simulink model "modelo_FunctionalArchitecture"  (R2021b)
settings: Solver=VariableStepAuto  StartTime=0.0  StopTime=10.0  RelTol=1e-3
settings Model: Creator=The MathWorks, Inc.  LastModifiedBy=David
settings SolverCC: AlgebraicLoopSolver=TrustRegion
settings DebuggingCC: SFMachineParentedDataDiag=warning

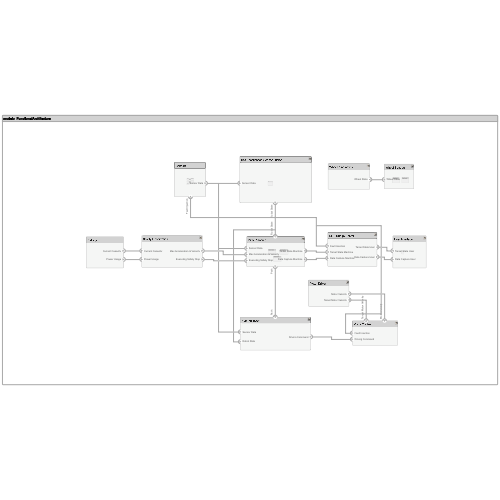
[thumbnail: Simulink's stored preview of the top-level diagram]
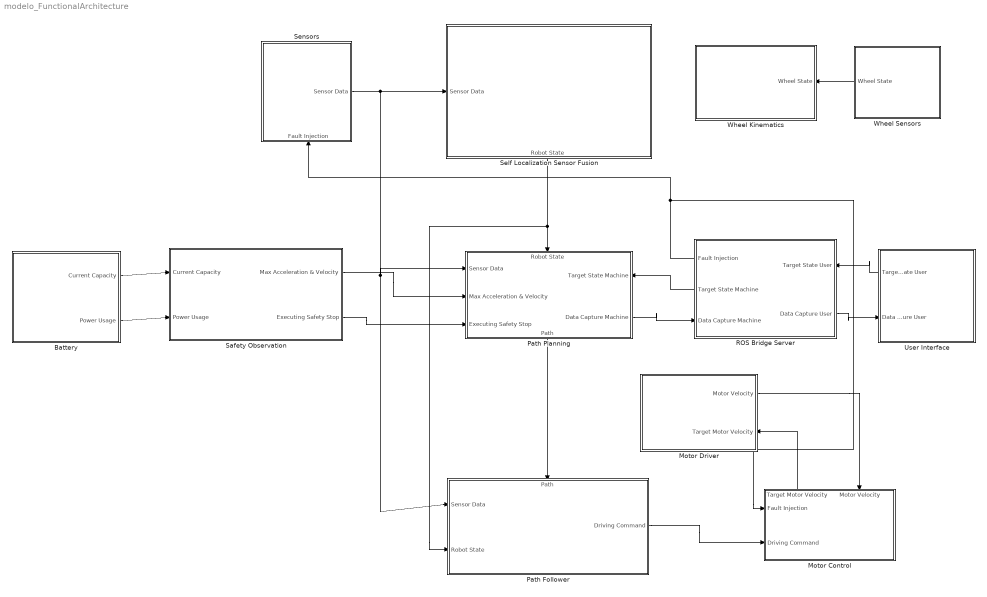
== system modelo_FunctionalArchitecture ==
  Battery : Subsystem
      settings: PortSchema="{\"entries\":[{\"content\":{\"headerSize\":26,\"margin\":15,\"minimumSpacing\":25,\"sides\":[{\"content\":{\"connectorIds\":[]},\"type\":\"ConnectorPlacement.EquallySpacedRectSide\",\"uuid\":\"59d5bf69-6351-4871-b6d0-e1e3e13a253a\"},{\"content\":{\"connectorIds\":[\"Out2\",\"Out1\"],\"side\":\"RIGHT\"},\"type\":\"ConnectorPlacement.EquallySpacedRectSide\",\"uuid\":\"4e75575f-31e6-4ae3-8223-3162d8144360\"},{\"content\":{\"connectorIds\":[],\"side\":\"TOP\"},\"type\":\"ConnectorPlacement.EquallySpacedRectSide\",\"uuid\":\"b9fd9e46-44c6-49b0-a9fa-d32b2dd616b0\"},{\"content\":{\"connectorIds\":[],\"side\":\"BOTTOM\"},\"type\":\"ConnectorPlacement.EquallySpacedRectSide\",\"uuid\":\"66421574-ce9c-483e-84db-c4bfc446eec2\"}]},\"type\":\"ConnectorPlacement.EquallySpacedConnector\",\"uuid\":\"4867c3fc-b41a-4efb-bf90-af290271d3df\"}],\"packageUris\":[\"http://schema.mathworks.com/mf0/Connector/R2020b\"],\"version\":\"1.0\"}"
  Motor Control : Subsystem
      settings: PortSchema="{\"entries\":[{\"content\":{\"headerSize\":26,\"margin\":15,\"minimumSpacing\":25,\"sides\":[{\"content\":{\"connectorIds\":[\"In1\",\"In3\"]},\"type\":\"ConnectorPlacement.EquallySpacedRectSide\",\"uuid\":\"59d5bf69-6351-4871-b6d0-e1e3e13a253a\"},{\"content\":{\"connectorIds\":[],\"side\":\"RIGHT\"},\"type\":\"ConnectorPlacement.EquallySpacedRectSide\",\"uuid\":\"4e75575f-31e6-4ae3-8223-3162d8144360\"},{\"content\":{\"connectorIds\":[\"Out1\",\"In2\"],\"side\":\"TOP\"},\"type\":\"ConnectorPlacement.EquallySpacedRectSide\",\"uuid\":\"b9fd9e46-44c6-49b0-a9fa-d32b2dd616b0\"}]},\"type\":\"ConnectorPlacement.EquallySpacedConnector\",\"uuid\":\"4867c3fc-b41a-4efb-bf90-af290271d3df\"}],\"packageUris\":[\"http://schema.mathworks.com/mf0/Connector/R2020b\"],\"version\":\"1.0\"}"
  Motor Driver : Subsystem
      settings: PortSchema="{\"entries\":[{\"content\":{\"headerSize\":26,\"margin\":15,\"minimumSpacing\":25,\"sides\":[{\"content\":{\"connectorIds\":[]},\"type\":\"ConnectorPlacement.EquallySpacedRectSide\",\"uuid\":\"59d5bf69-6351-4871-b6d0-e1e3e13a253a\"},{\"content\":{\"connectorIds\":[\"Out1\",\"In1\"],\"side\":\"RIGHT\"},\"type\":\"ConnectorPlacement.EquallySpacedRectSide\",\"uuid\":\"4e75575f-31e6-4ae3-8223-3162d8144360\"},{\"content\":{\"connectorIds\":[],\"side\":\"TOP\"},\"type\":\"ConnectorPlacement.EquallySpacedRectSide\",\"uuid\":\"b9fd9e46-44c6-49b0-a9fa-d32b2dd616b0\"},{\"content\":{\"connectorIds\":[],\"side\":\"BOTTOM\"},\"type\":\"ConnectorPlacement.EquallySpacedRectSide\",\"uuid\":\"67d81e08-878d-4ffc-8e69-7bb62ac9563c\"}]},\"type\":\"ConnectorPlacement.EquallySpacedConnector\",\"uuid\":\"4867c3fc-b41a-4efb-bf90-af290271d3df\"}],\"packageUris\":[\"http://schema.mathworks.com/mf0/Connector/R2020b\"],\"version\":\"1.0\"}"
  Path Follower : Subsystem
      settings: PortSchema="{\"entries\":[{\"content\":{\"headerSize\":26,\"margin\":15,\"minimumSpacing\":25,\"sides\":[{\"content\":{\"connectorIds\":[\"In1\",\"In3\"]},\"type\":\"ConnectorPlacement.EquallySpacedRectSide\",\"uuid\":\"59d5bf69-6351-4871-b6d0-e1e3e13a253a\"},{\"content\":{\"connectorIds\":[\"Out1\"],\"side\":\"RIGHT\"},\"type\":\"ConnectorPlacement.EquallySpacedRectSide\",\"uuid\":\"4e75575f-31e6-4ae3-8223-3162d8144360\"},{\"content\":{\"connectorIds\":[\"In2\"],\"side\":\"TOP\"},\"type\":\"ConnectorPlacement.EquallySpacedRectSide\",\"uuid\":\"b9fd9e46-44c6-49b0-a9fa-d32b2dd616b0\"}]},\"type\":\"ConnectorPlacement.EquallySpacedConnector\",\"uuid\":\"4867c3fc-b41a-4efb-bf90-af290271d3df\"}],\"packageUris\":[\"http://schema.mathworks.com/mf0/Connector/R2020b\"],\"version\":\"1.0\"}"
  Path Planning : Subsystem
      settings: PortSchema="{\"entries\":[{\"content\":{\"headerSize\":26,\"margin\":15,\"minimumSpacing\":25,\"sides\":[{\"content\":{\"connectorIds\":[\"In1\",\"In2\",\"In3\"]},\"type\":\"ConnectorPlacement.EquallySpacedRectSide\",\"uuid\":\"59d5bf69-6351-4871-b6d0-e1e3e13a253a\"},{\"content\":{\"connectorIds\":[\"In4\",\"Out1\"],\"side\":\"RIGHT\"},\"type\":\"ConnectorPlacement.EquallySpacedRectSide\",\"uuid\":\"4e75575f-31e6-4ae3-8223-3162d8144360\"},{\"content\":{\"connectorIds\":[\"In5\"],\"side\":\"TOP\"},\"type\":\"ConnectorPlacement.EquallySpacedRectSide\",\"uuid\":\"b9fd9e46-44c6-49b0-a9fa-d32b2dd616b0\"},{\"content\":{\"connectorIds\":[\"Out2\"],\"side\":\"BOTTOM\"},\"type\":\"ConnectorPlacement.EquallySpacedRectSide\",\"uuid\":\"b63bab7c-787a-46d6-b750-862a2a39c4b0\"}]},\"type\":\"ConnectorPlacement.EquallySpacedConnector\",\"uuid\":\"4867c3fc-b41a-4efb-bf90-af290271d3df\"}],\"packageUris\":[\"http://schema.mathworks.com/mf0/Connector/R2020b\"],\"version\":\"1.0\"}"
  ROS Bridge Server : Subsystem
      settings: PortSchema="{\"entries\":[{\"content\":{\"headerSize\":26,\"margin\":15,\"minimumSpacing\":25,\"sides\":[{\"content\":{\"connectorIds\":[\"Out1\",\"Out3\",\"In1\"]},\"type\":\"ConnectorPlacement.EquallySpacedRectSide\",\"uuid\":\"78ec9596-c19b-4a19-90cc-d79d904dcecb\"},{\"content\":{\"connectorIds\":[\"In2\",\"Out2\"],\"side\":\"RIGHT\"},\"type\":\"ConnectorPlacement.EquallySpacedRectSide\",\"uuid\":\"e50c32f8-61a1-4c3e-810e-7c092ec61b9d\"},{\"content\":{\"connectorIds\":[],\"side\":\"TOP\"},\"type\":\"ConnectorPlacement.EquallySpacedRectSide\",\"uuid\":\"dd5589de-c446-44bc-b6c3-43d178c94f81\"}]},\"type\":\"ConnectorPlacement.EquallySpacedConnector\",\"uuid\":\"1e9f716a-1f22-4423-b94e-8264810d47f5\"}],\"packageUris\":[\"http://schema.mathworks.com/mf0/Connector/R2020b\"],\"version\":\"1.0\"}"
  Safety Observation : Subsystem
      settings: PortSchema="{\"entries\":[{\"content\":{\"headerSize\":26,\"margin\":15,\"minimumSpacing\":25,\"sides\":[{\"content\":{\"connectorIds\":[\"In2\",\"In1\"]},\"type\":\"ConnectorPlacement.EquallySpacedRectSide\",\"uuid\":\"59d5bf69-6351-4871-b6d0-e1e3e13a253a\"},{\"content\":{\"connectorIds\":[\"Out2\",\"Out1\"],\"side\":\"RIGHT\"},\"type\":\"ConnectorPlacement.EquallySpacedRectSide\",\"uuid\":\"4e75575f-31e6-4ae3-8223-3162d8144360\"},{\"content\":{\"connectorIds\":[],\"side\":\"TOP\"},\"type\":\"ConnectorPlacement.EquallySpacedRectSide\",\"uuid\":\"b9fd9e46-44c6-49b0-a9fa-d32b2dd616b0\"},{\"content\":{\"connectorIds\":[],\"side\":\"BOTTOM\"},\"type\":\"ConnectorPlacement.EquallySpacedRectSide\",\"uuid\":\"4263e838-8ece-4353-a266-fb02fc9beff8\"}]},\"type\":\"ConnectorPlacement.EquallySpacedConnector\",\"uuid\":\"4867c3fc-b41a-4efb-bf90-af290271d3df\"}],\"packageUris\":[\"http://schema.mathworks.com/mf0/Connector/R2020b\"],\"version\":\"1.0\"}"
  Self Localization Sensor Fusion : Subsystem
      settings: PortSchema="{\"entries\":[{\"content\":{\"headerSize\":26,\"margin\":15,\"minimumSpacing\":25,\"sides\":[{\"content\":{\"connectorIds\":[\"In1\"]},\"type\":\"ConnectorPlacement.EquallySpacedRectSide\",\"uuid\":\"59d5bf69-6351-4871-b6d0-e1e3e13a253a\"},{\"content\":{\"connectorIds\":[],\"side\":\"RIGHT\"},\"type\":\"ConnectorPlacement.EquallySpacedRectSide\",\"uuid\":\"4e75575f-31e6-4ae3-8223-3162d8144360\"},{\"content\":{\"connectorIds\":[],\"side\":\"TOP\"},\"type\":\"ConnectorPlacement.EquallySpacedRectSide\",\"uuid\":\"b9fd9e46-44c6-49b0-a9fa-d32b2dd616b0\"},{\"content\":{\"connectorIds\":[\"Out1\"],\"side\":\"BOTTOM\"},\"type\":\"ConnectorPlacement.EquallySpacedRectSide\",\"uuid\":\"114bac9a-6c92-45bb-ae46-c4bda2c799d1\"}]},\"type\":\"ConnectorPlacement.EquallySpacedConnector\",\"uuid\":\"4867c3fc-b41a-4efb-bf90-af290271d3df\"}],\"packageUris\":[\"http://schema.mathworks.com/mf0/Connector/R2020b\"],\"version\":\"1.0\"}"
  Sensors : Subsystem
      settings: PortSchema="{\"entries\":[{\"content\":{\"headerSize\":26,\"margin\":15,\"minimumSpacing\":25,\"sides\":[{\"content\":{\"connectorIds\":[]},\"type\":\"ConnectorPlacement.EquallySpacedRectSide\",\"uuid\":\"78ec9596-c19b-4a19-90cc-d79d904dcecb\"},{\"content\":{\"connectorIds\":[\"Out1\"],\"side\":\"RIGHT\"},\"type\":\"ConnectorPlacement.EquallySpacedRectSide\",\"uuid\":\"e50c32f8-61a1-4c3e-810e-7c092ec61b9d\"},{\"content\":{\"connectorIds\":[],\"side\":\"TOP\"},\"type\":\"ConnectorPlacement.EquallySpacedRectSide\",\"uuid\":\"dd5589de-c446-44bc-b6c3-43d178c94f81\"},{\"content\":{\"connectorIds\":[\"In1\"],\"side\":\"BOTTOM\"},\"type\":\"ConnectorPlacement.EquallySpacedRectSide\",\"uuid\":\"022d1208-42d8-4ed3-aa9f-a16a2de5d603\"}]},\"type\":\"ConnectorPlacement.EquallySpacedConnector\",\"uuid\":\"1e9f716a-1f22-4423-b94e-8264810d47f5\"}],\"packageUris\":[\"http://schema.mathworks.com/mf0/Connector/R2020b\"],\"version\":\"1.0\"}"
  User Interface : Subsystem
      settings: PortSchema="{\"entries\":[{\"content\":{\"headerSize\":26,\"margin\":15,\"minimumSpacing\":25,\"sides\":[{\"content\":{\"connectorIds\":[\"Out1\",\"In1\"]},\"type\":\"ConnectorPlacement.EquallySpacedRectSide\",\"uuid\":\"59d5bf69-6351-4871-b6d0-e1e3e13a253a\"},{\"content\":{\"connectorIds\":[],\"side\":\"RIGHT\"},\"type\":\"ConnectorPlacement.EquallySpacedRectSide\",\"uuid\":\"4e75575f-31e6-4ae3-8223-3162d8144360\"},{\"content\":{\"connectorIds\":[],\"side\":\"TOP\"},\"type\":\"ConnectorPlacement.EquallySpacedRectSide\",\"uuid\":\"b9fd9e46-44c6-49b0-a9fa-d32b2dd616b0\"},{\"content\":{\"connectorIds\":[],\"side\":\"BOTTOM\"},\"type\":\"ConnectorPlacement.EquallySpacedRectSide\",\"uuid\":\"51492fe5-00fa-4995-98e1-4969e22079d3\"}]},\"type\":\"ConnectorPlacement.EquallySpacedConnector\",\"uuid\":\"4867c3fc-b41a-4efb-bf90-af290271d3df\"}],\"packageUris\":[\"http://schema.mathworks.com/mf0/Connector/R2020b\"],\"version\":\"1.0\"}"
  Wheel Kinematics : Subsystem
      settings: PortSchema="{\"entries\":[{\"content\":{\"headerSize\":26,\"margin\":15,\"minimumSpacing\":25,\"sides\":[{\"content\":{\"connectorIds\":[]},\"type\":\"ConnectorPlacement.EquallySpacedRectSide\",\"uuid\":\"8b00e6c1-78bc-425f-98b4-5345e91b6ef3\"},{\"content\":{\"connectorIds\":[\"In1\"],\"side\":\"RIGHT\"},\"type\":\"ConnectorPlacement.EquallySpacedRectSide\",\"uuid\":\"cca7f40b-c9e3-40f8-88e3-c95e453373a7\"},{\"content\":{\"connectorIds\":[],\"side\":\"TOP\"},\"type\":\"ConnectorPlacement.EquallySpacedRectSide\",\"uuid\":\"2cebc568-363b-44c7-85e9-8321d53d58f8\"}]},\"type\":\"ConnectorPlacement.EquallySpacedConnector\",\"uuid\":\"893f8d0c-b80d-487c-8abd-26601278087d\"}],\"packageUris\":[\"http://schema.mathworks.com/mf0/Connector/R2020b\"],\"version\":\"1.0\"}"
  Wheel Sensors : Subsystem
      settings: PortSchema="{\"entries\":[{\"content\":{\"headerSize\":26,\"margin\":15,\"minimumSpacing\":25,\"sides\":[{\"content\":{\"connectorIds\":[\"Out1\"]},\"type\":\"ConnectorPlacement.EquallySpacedRectSide\",\"uuid\":\"59d5bf69-6351-4871-b6d0-e1e3e13a253a\"},{\"content\":{\"connectorIds\":[],\"side\":\"RIGHT\"},\"type\":\"ConnectorPlacement.EquallySpacedRectSide\",\"uuid\":\"4e75575f-31e6-4ae3-8223-3162d8144360\"},{\"content\":{\"connectorIds\":[],\"side\":\"TOP\"},\"type\":\"ConnectorPlacement.EquallySpacedRectSide\",\"uuid\":\"b9fd9e46-44c6-49b0-a9fa-d32b2dd616b0\"}]},\"type\":\"ConnectorPlacement.EquallySpacedConnector\",\"uuid\":\"4867c3fc-b41a-4efb-bf90-af290271d3df\"}],\"packageUris\":[\"http://schema.mathworks.com/mf0/Connector/R2020b\"],\"version\":\"1.0\"}"
  wires:
  Self Localization Sensor Fusion/1(Robot State) -> Path Follower/3(Robot State), Path Planning/5(Robot State)
  Safety Observation/2(Max Acceleration & Velocity) -> Path Planning/2(Max Acceleration & Velocity)
  Path Follower/1(Driving Command) -> Motor Control/3(Driving Command)
  Battery/1(Power Usage) -> Safety Observation/1(Power Usage)
  Battery/2(Current Capacity) -> Safety Observation/2(Current Capacity)
  Motor Driver/1(Motor Velocity) -> Motor Control/2(Motor Velocity)
  Motor Control/1(Target Motor Velocity) -> Motor Driver/1(Target Motor Velocity)
  Path Planning/2(Path) -> Path Follower/2(Path)
  Safety Observation/1(Executing Safety Stop) -> Path Planning/3(Executing Safety Stop)
  Wheel Sensors/1(Wheel State) -> Wheel Kinematics/1(Wheel State)
  User Interface/1(Target State User) -> ROS Bridge Server/2(Target State User)
  ROS Bridge Server/3(Target State Machine) -> Path Planning/4(Target State Machine)
  Path Planning/1(Data Capture Machine) -> ROS Bridge Server/1(Data Capture Machine)
  ROS Bridge Server/2(Data Capture User) -> User Interface/1(Data Capture User)
  Sensors/1(Sensor Data) -> Path Follower/1(Sensor Data), Path Planning/1(Sensor Data), Self Localization Sensor Fusion/1(Sensor Data)
  ROS Bridge Server/1(Fault Injection) -> Motor Control/1(Fault Injection), Sensors/1(Fault Injection)

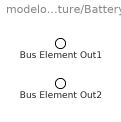
== system modelo_FunctionalArchitecture/Battery ==
  Bus Element Out1 : Outport  PortName=Power Usage
  Bus Element Out2 : Outport  Port=2  PortName=Current Capacity

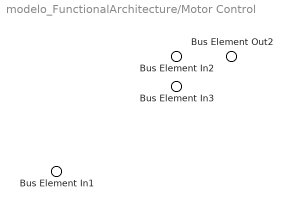
== system modelo_FunctionalArchitecture/Motor Control ==
  Bus Element In3 : Inport  PortName=Fault Injection
  Bus Element In2 : Inport  Port=2  PortName=Motor Velocity
  Bus Element In1 : Inport  Port=3  PortName=Driving Command
  Bus Element Out2 : Outport  PortName=Target Motor Velocity

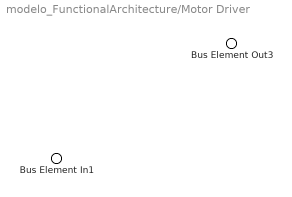
== system modelo_FunctionalArchitecture/Motor Driver ==
  Bus Element In1 : Inport  PortName=Target Motor Velocity
  Bus Element Out3 : Outport  PortName=Motor Velocity

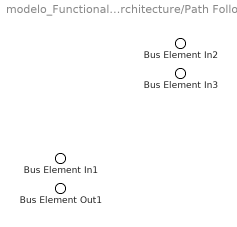
== system modelo_FunctionalArchitecture/Path Follower ==
  Bus Element In2 : Inport  PortName=Sensor Data
  Bus Element In3 : Inport  Port=2  PortName=Path
  Bus Element In1 : Inport  Port=3  PortName=Robot State
  Bus Element Out1 : Outport  PortName=Driving Command

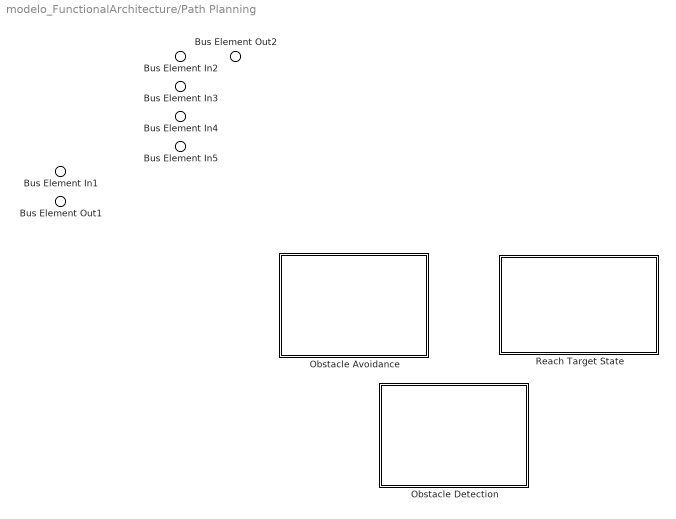
== system modelo_FunctionalArchitecture/Path Planning ==
  Bus Element In3 : Inport  PortName=Sensor Data
  Bus Element In4 : Inport  Port=2  PortName=Max Acceleration & Velocity
  Bus Element In5 : Inport  Port=3  PortName=Executing Safety Stop
  Bus Element In2 : Inport  Port=4  PortName=Target State Machine
  Bus Element In1 : Inport  Port=5  PortName=Robot State
  Obstacle Avoidance : Subsystem
      settings: PortSchema="{\"entries\":[{\"content\":{\"headerSize\":26,\"margin\":15,\"minimumSpacing\":25,\"sides\":[{\"content\":{\"connectorIds\":[]},\"type\":\"ConnectorPlacement.EquallySpacedRectSide\",\"uuid\":\"623c0a04-b13a-4ec6-8a7d-dfc6306469bc\"},{\"content\":{\"connectorIds\":[],\"side\":\"RIGHT\"},\"type\":\"ConnectorPlacement.EquallySpacedRectSide\",\"uuid\":\"78f920bb-0077-4b2a-aa3f-2f201c60998f\"},{\"content\":{\"connectorIds\":[],\"side\":\"TOP\"},\"type\":\"ConnectorPlacement.EquallySpacedRectSide\",\"uuid\":\"9b1e3f50-ee79-4c39-a86a-2d702aea3294\"},{\"content\":{\"connectorIds\":[],\"side\":\"HIDDEN\"},\"type\":\"ConnectorPlacement.EquallySpacedRectSide\",\"uuid\":\"cdf686db-25c9-46dd-b452-4d2a5526d98f\"}]},\"type\":\"ConnectorPlacement.EquallySpacedConnector\",\"uuid\":\"0b3e7296-fe8f-4ed3-b294-7805e2066d7f\"}],\"packageUris\":[\"http://schema.mathworks.com/mf0/Connector/R2020b\"],\"version\":\"1.0\"}"
  Obstacle Detection : Subsystem
      settings: PortSchema="{\"entries\":[{\"content\":{\"headerSize\":26,\"margin\":15,\"minimumSpacing\":25,\"sides\":[{\"content\":{\"connectorIds\":[]},\"type\":\"ConnectorPlacement.EquallySpacedRectSide\",\"uuid\":\"623c0a04-b13a-4ec6-8a7d-dfc6306469bc\"},{\"content\":{\"connectorIds\":[],\"side\":\"RIGHT\"},\"type\":\"ConnectorPlacement.EquallySpacedRectSide\",\"uuid\":\"78f920bb-0077-4b2a-aa3f-2f201c60998f\"},{\"content\":{\"connectorIds\":[],\"side\":\"TOP\"},\"type\":\"ConnectorPlacement.EquallySpacedRectSide\",\"uuid\":\"9b1e3f50-ee79-4c39-a86a-2d702aea3294\"},{\"content\":{\"connectorIds\":[],\"side\":\"HIDDEN\"},\"type\":\"ConnectorPlacement.EquallySpacedRectSide\",\"uuid\":\"cdf686db-25c9-46dd-b452-4d2a5526d98f\"}]},\"type\":\"ConnectorPlacement.EquallySpacedConnector\",\"uuid\":\"0b3e7296-fe8f-4ed3-b294-7805e2066d7f\"}],\"packageUris\":[\"http://schema.mathworks.com/mf0/Connector/R2020b\"],\"version\":\"1.0\"}"
  Reach Target State : Subsystem
      settings: PortSchema="{\"entries\":[{\"content\":{\"headerSize\":26,\"margin\":15,\"minimumSpacing\":25,\"sides\":[{\"content\":{\"connectorIds\":[]},\"type\":\"ConnectorPlacement.EquallySpacedRectSide\",\"uuid\":\"623c0a04-b13a-4ec6-8a7d-dfc6306469bc\"},{\"content\":{\"connectorIds\":[],\"side\":\"RIGHT\"},\"type\":\"ConnectorPlacement.EquallySpacedRectSide\",\"uuid\":\"78f920bb-0077-4b2a-aa3f-2f201c60998f\"},{\"content\":{\"connectorIds\":[],\"side\":\"TOP\"},\"type\":\"ConnectorPlacement.EquallySpacedRectSide\",\"uuid\":\"9b1e3f50-ee79-4c39-a86a-2d702aea3294\"},{\"content\":{\"connectorIds\":[],\"side\":\"HIDDEN\"},\"type\":\"ConnectorPlacement.EquallySpacedRectSide\",\"uuid\":\"cdf686db-25c9-46dd-b452-4d2a5526d98f\"}]},\"type\":\"ConnectorPlacement.EquallySpacedConnector\",\"uuid\":\"0b3e7296-fe8f-4ed3-b294-7805e2066d7f\"}],\"packageUris\":[\"http://schema.mathworks.com/mf0/Connector/R2020b\"],\"version\":\"1.0\"}"
  Bus Element Out2 : Outport  PortName=Data Capture Machine
  Bus Element Out1 : Outport  Port=2  PortName=Path

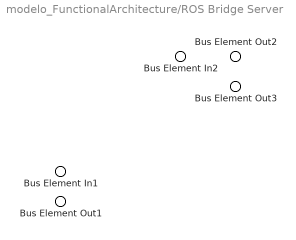
== system modelo_FunctionalArchitecture/ROS Bridge Server ==
  Bus Element In2 : Inport  PortName=Data Capture Machine
  Bus Element In1 : Inport  Port=2  PortName=Target State User
  Bus Element Out3 : Outport  PortName=Fault Injection
  Bus Element Out2 : Outport  Port=2  PortName=Data Capture User
  Bus Element Out1 : Outport  Port=3  PortName=Target State Machine

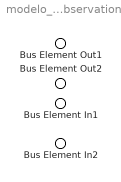
== system modelo_FunctionalArchitecture/Safety Observation ==
  Bus Element In1 : Inport  PortName=Power Usage
  Bus Element In2 : Inport  Port=2  PortName=Current Capacity
  Bus Element Out1 : Outport  PortName=Executing Safety Stop
  Bus Element Out2 : Outport  Port=2  PortName=Max Acceleration & Velocity

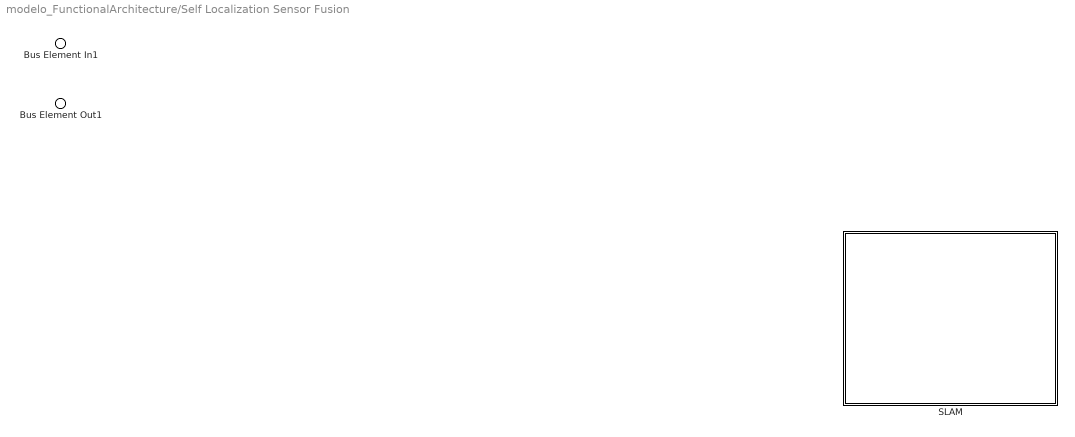
== system modelo_FunctionalArchitecture/Self Localization Sensor Fusion ==
  Bus Element In1 : Inport  PortName=Sensor Data
  SLAM : Subsystem
      settings: PortSchema="{\"entries\":[{\"content\":{\"headerSize\":26,\"margin\":15,\"minimumSpacing\":25,\"sides\":[{\"content\":{\"connectorIds\":[]},\"type\":\"ConnectorPlacement.EquallySpacedRectSide\",\"uuid\":\"78ec9596-c19b-4a19-90cc-d79d904dcecb\"},{\"content\":{\"connectorIds\":[],\"side\":\"RIGHT\"},\"type\":\"ConnectorPlacement.EquallySpacedRectSide\",\"uuid\":\"e50c32f8-61a1-4c3e-810e-7c092ec61b9d\"},{\"content\":{\"connectorIds\":[],\"side\":\"TOP\"},\"type\":\"ConnectorPlacement.EquallySpacedRectSide\",\"uuid\":\"dd5589de-c446-44bc-b6c3-43d178c94f81\"}]},\"type\":\"ConnectorPlacement.EquallySpacedConnector\",\"uuid\":\"1e9f716a-1f22-4423-b94e-8264810d47f5\"}],\"packageUris\":[\"http://schema.mathworks.com/mf0/Connector/R2020b\"],\"version\":\"1.0\"}"
  Bus Element Out1 : Outport  PortName=Robot State

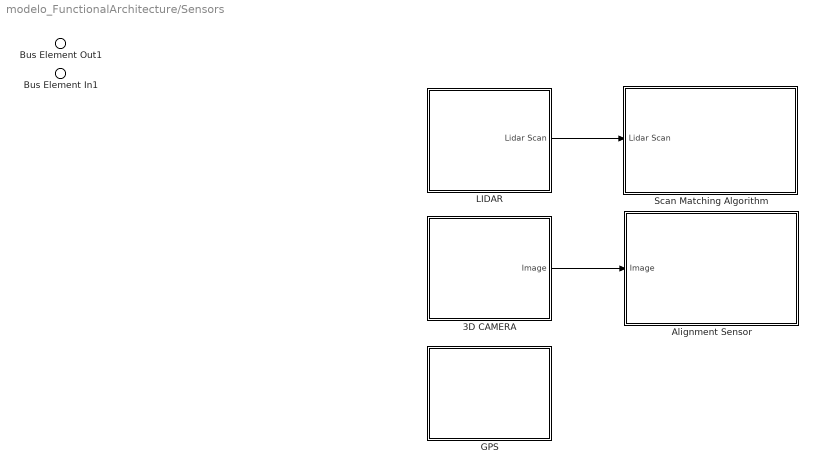
== system modelo_FunctionalArchitecture/Sensors ==
  Bus Element In1 : Inport  PortName=Fault Injection
  3D CAMERA : Subsystem
      settings: PortSchema="{\"entries\":[{\"content\":{\"headerSize\":26,\"margin\":15,\"minimumSpacing\":25,\"sides\":[{\"content\":{\"connectorIds\":[]},\"type\":\"ConnectorPlacement.EquallySpacedRectSide\",\"uuid\":\"8b00e6c1-78bc-425f-98b4-5345e91b6ef3\"},{\"content\":{\"connectorIds\":[\"Out1\"],\"side\":\"RIGHT\"},\"type\":\"ConnectorPlacement.EquallySpacedRectSide\",\"uuid\":\"cca7f40b-c9e3-40f8-88e3-c95e453373a7\"},{\"content\":{\"connectorIds\":[],\"side\":\"TOP\"},\"type\":\"ConnectorPlacement.EquallySpacedRectSide\",\"uuid\":\"2cebc568-363b-44c7-85e9-8321d53d58f8\"}]},\"type\":\"ConnectorPlacement.EquallySpacedConnector\",\"uuid\":\"893f8d0c-b80d-487c-8abd-26601278087d\"}],\"packageUris\":[\"http://schema.mathworks.com/mf0/Connector/R2020b\"],\"version\":\"1.0\"}"
  Alignment Sensor : Subsystem
      settings: PortSchema="{\"entries\":[{\"content\":{\"headerSize\":26,\"margin\":15,\"minimumSpacing\":25,\"sides\":[{\"content\":{\"connectorIds\":[\"In1\"]},\"type\":\"ConnectorPlacement.EquallySpacedRectSide\",\"uuid\":\"8b00e6c1-78bc-425f-98b4-5345e91b6ef3\"},{\"content\":{\"connectorIds\":[],\"side\":\"RIGHT\"},\"type\":\"ConnectorPlacement.EquallySpacedRectSide\",\"uuid\":\"cca7f40b-c9e3-40f8-88e3-c95e453373a7\"},{\"content\":{\"connectorIds\":[],\"side\":\"TOP\"},\"type\":\"ConnectorPlacement.EquallySpacedRectSide\",\"uuid\":\"2cebc568-363b-44c7-85e9-8321d53d58f8\"}]},\"type\":\"ConnectorPlacement.EquallySpacedConnector\",\"uuid\":\"893f8d0c-b80d-487c-8abd-26601278087d\"}],\"packageUris\":[\"http://schema.mathworks.com/mf0/Connector/R2020b\"],\"version\":\"1.0\"}"
  GPS : Subsystem
      settings: PortSchema="{\"entries\":[{\"content\":{\"headerSize\":26,\"margin\":15,\"minimumSpacing\":25,\"sides\":[{\"content\":{\"connectorIds\":[]},\"type\":\"ConnectorPlacement.EquallySpacedRectSide\",\"uuid\":\"78ec9596-c19b-4a19-90cc-d79d904dcecb\"},{\"content\":{\"connectorIds\":[],\"side\":\"RIGHT\"},\"type\":\"ConnectorPlacement.EquallySpacedRectSide\",\"uuid\":\"e50c32f8-61a1-4c3e-810e-7c092ec61b9d\"},{\"content\":{\"connectorIds\":[],\"side\":\"TOP\"},\"type\":\"ConnectorPlacement.EquallySpacedRectSide\",\"uuid\":\"dd5589de-c446-44bc-b6c3-43d178c94f81\"}]},\"type\":\"ConnectorPlacement.EquallySpacedConnector\",\"uuid\":\"1e9f716a-1f22-4423-b94e-8264810d47f5\"}],\"packageUris\":[\"http://schema.mathworks.com/mf0/Connector/R2020b\"],\"version\":\"1.0\"}"
  LIDAR : Subsystem
      settings: PortSchema="{\"entries\":[{\"content\":{\"headerSize\":26,\"margin\":15,\"minimumSpacing\":25,\"sides\":[{\"content\":{\"connectorIds\":[]},\"type\":\"ConnectorPlacement.EquallySpacedRectSide\",\"uuid\":\"59d5bf69-6351-4871-b6d0-e1e3e13a253a\"},{\"content\":{\"connectorIds\":[\"Out1\"],\"side\":\"RIGHT\"},\"type\":\"ConnectorPlacement.EquallySpacedRectSide\",\"uuid\":\"4e75575f-31e6-4ae3-8223-3162d8144360\"},{\"content\":{\"connectorIds\":[],\"side\":\"TOP\"},\"type\":\"ConnectorPlacement.EquallySpacedRectSide\",\"uuid\":\"b9fd9e46-44c6-49b0-a9fa-d32b2dd616b0\"}]},\"type\":\"ConnectorPlacement.EquallySpacedConnector\",\"uuid\":\"4867c3fc-b41a-4efb-bf90-af290271d3df\"}],\"packageUris\":[\"http://schema.mathworks.com/mf0/Connector/R2020b\"],\"version\":\"1.0\"}"
  Scan Matching Algorithm : Subsystem
      settings: PortSchema="{\"entries\":[{\"content\":{\"headerSize\":26,\"margin\":15,\"minimumSpacing\":25,\"sides\":[{\"content\":{\"connectorIds\":[\"In1\"]},\"type\":\"ConnectorPlacement.EquallySpacedRectSide\",\"uuid\":\"8b00e6c1-78bc-425f-98b4-5345e91b6ef3\"},{\"content\":{\"connectorIds\":[],\"side\":\"RIGHT\"},\"type\":\"ConnectorPlacement.EquallySpacedRectSide\",\"uuid\":\"cca7f40b-c9e3-40f8-88e3-c95e453373a7\"},{\"content\":{\"connectorIds\":[],\"side\":\"TOP\"},\"type\":\"ConnectorPlacement.EquallySpacedRectSide\",\"uuid\":\"2cebc568-363b-44c7-85e9-8321d53d58f8\"}]},\"type\":\"ConnectorPlacement.EquallySpacedConnector\",\"uuid\":\"893f8d0c-b80d-487c-8abd-26601278087d\"}],\"packageUris\":[\"http://schema.mathworks.com/mf0/Connector/R2020b\"],\"version\":\"1.0\"}"
  Bus Element Out1 : Outport  PortName=Sensor Data
  wires:
  3D CAMERA/1(Image) -> Alignment Sensor/1(Image)
  LIDAR/1(Lidar Scan) -> Scan Matching Algorithm/1(Lidar Scan)

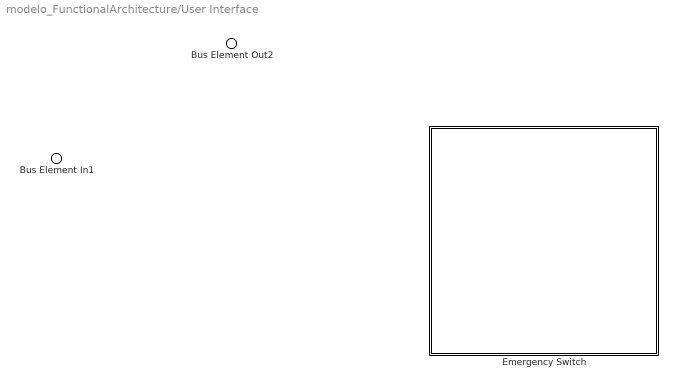
== system modelo_FunctionalArchitecture/User Interface ==
  Bus Element In1 : Inport  PortName=Data Capture User
  Emergency Switch : Subsystem
      settings: PortSchema="{\"entries\":[{\"content\":{\"headerSize\":26,\"margin\":15,\"minimumSpacing\":25,\"sides\":[{\"content\":{\"connectorIds\":[]},\"type\":\"ConnectorPlacement.EquallySpacedRectSide\",\"uuid\":\"78ec9596-c19b-4a19-90cc-d79d904dcecb\"},{\"content\":{\"connectorIds\":[],\"side\":\"RIGHT\"},\"type\":\"ConnectorPlacement.EquallySpacedRectSide\",\"uuid\":\"e50c32f8-61a1-4c3e-810e-7c092ec61b9d\"},{\"content\":{\"connectorIds\":[],\"side\":\"TOP\"},\"type\":\"ConnectorPlacement.EquallySpacedRectSide\",\"uuid\":\"dd5589de-c446-44bc-b6c3-43d178c94f81\"}]},\"type\":\"ConnectorPlacement.EquallySpacedConnector\",\"uuid\":\"1e9f716a-1f22-4423-b94e-8264810d47f5\"}],\"packageUris\":[\"http://schema.mathworks.com/mf0/Connector/R2020b\"],\"version\":\"1.0\"}"
  Bus Element Out2 : Outport  PortName=Target State User

== system modelo_FunctionalArchitecture/Wheel Kinematics ==
  Bus Element In1 : Inport  PortName=Wheel State

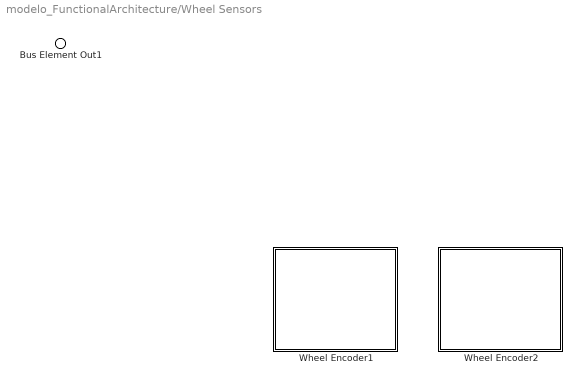
== system modelo_FunctionalArchitecture/Wheel Sensors ==
  Wheel Encoder1 : Subsystem
      settings: PortSchema="{\"entries\":[{\"content\":{\"headerSize\":26,\"margin\":15,\"minimumSpacing\":25,\"sides\":[{\"content\":{\"connectorIds\":[]},\"type\":\"ConnectorPlacement.EquallySpacedRectSide\",\"uuid\":\"6da287f1-0145-4984-81ce-516f9d473d08\"},{\"content\":{\"connectorIds\":[],\"side\":\"RIGHT\"},\"type\":\"ConnectorPlacement.EquallySpacedRectSide\",\"uuid\":\"e8258003-a16e-4667-bad1-2432c305b2b4\"},{\"content\":{\"connectorIds\":[],\"side\":\"TOP\"},\"type\":\"ConnectorPlacement.EquallySpacedRectSide\",\"uuid\":\"774c20e3-3d70-4446-b47a-ebbe701b6bb4\"}]},\"type\":\"ConnectorPlacement.EquallySpacedConnector\",\"uuid\":\"18cfb653-cd4a-4ba6-a2cf-b79d05bb2a8a\"}],\"packageUris\":[\"http://schema.mathworks.com/mf0/Connector/R2020b\"],\"version\":\"1.0\"}"
  Wheel Encoder2 : Subsystem
      settings: PortSchema="{\"entries\":[{\"content\":{\"headerSize\":26,\"margin\":15,\"minimumSpacing\":25,\"sides\":[{\"content\":{\"connectorIds\":[]},\"type\":\"ConnectorPlacement.EquallySpacedRectSide\",\"uuid\":\"6da287f1-0145-4984-81ce-516f9d473d08\"},{\"content\":{\"connectorIds\":[],\"side\":\"RIGHT\"},\"type\":\"ConnectorPlacement.EquallySpacedRectSide\",\"uuid\":\"e8258003-a16e-4667-bad1-2432c305b2b4\"},{\"content\":{\"connectorIds\":[],\"side\":\"TOP\"},\"type\":\"ConnectorPlacement.EquallySpacedRectSide\",\"uuid\":\"774c20e3-3d70-4446-b47a-ebbe701b6bb4\"}]},\"type\":\"ConnectorPlacement.EquallySpacedConnector\",\"uuid\":\"18cfb653-cd4a-4ba6-a2cf-b79d05bb2a8a\"}],\"packageUris\":[\"http://schema.mathworks.com/mf0/Connector/R2020b\"],\"version\":\"1.0\"}"
  Bus Element Out1 : Outport  PortName=Wheel State

== system modelo_FunctionalArchitecture/Path Planning/Obstacle Avoidance ==

== system modelo_FunctionalArchitecture/Path Planning/Obstacle Detection ==

== system modelo_FunctionalArchitecture/Path Planning/Reach Target State ==

== system modelo_FunctionalArchitecture/Self Localization Sensor Fusion/SLAM ==

== system modelo_FunctionalArchitecture/Sensors/3D CAMERA ==
  Bus Element Out1 : Outport  PortName=Image

== system modelo_FunctionalArchitecture/Sensors/Alignment Sensor ==
  Bus Element In1 : Inport  PortName=Image

== system modelo_FunctionalArchitecture/Sensors/GPS ==

== system modelo_FunctionalArchitecture/Sensors/LIDAR ==
  Bus Element Out1 : Outport  PortName=Lidar Scan

== system modelo_FunctionalArchitecture/Sensors/Scan Matching Algorithm ==
  Bus Element In1 : Inport  PortName=Lidar Scan

== system modelo_FunctionalArchitecture/User Interface/Emergency Switch ==

== system modelo_FunctionalArchitecture/Wheel Sensors/Wheel Encoder1 ==

== system modelo_FunctionalArchitecture/Wheel Sensors/Wheel Encoder2 ==
